simulink library "SCAN"  (R2016a)
settings: Solver=ode45  StartTime=0.0  StopTime=10.0  RelTol=1e-3
undefined symbols (not defined in the file): BLOCK_SIZE
settings Model: Creator=oelkawok  LastModifiedBy=oelkawok
settings DataIOCC: LimitDataPoints=on
settings DebuggingCC: AllowSymbolicDim=off

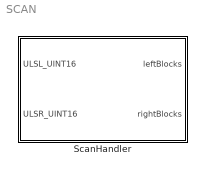
== system SCAN ==
  ScanHandler : Subsystem

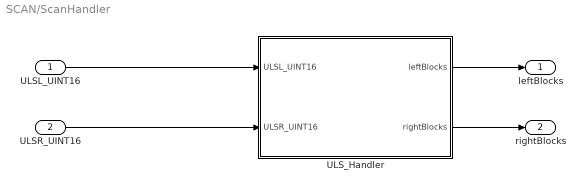
== system SCAN/ScanHandler ==
  ULSL_UINT16 : Inport  OutDataTypeStr=uint16  PortDimensions=1  SampleTime=[0.0050000000000000001,0]
  ULSR_UINT16 : Inport  Port=2  OutDataTypeStr=uint16  PortDimensions=1  SampleTime=[0.0050000000000000001,0]
  ULS_Handler : Subsystem
  leftBlocks : Outport
  rightBlocks : Outport  Port=2
  wires:
  ULSL_UINT16/1 -> ULS_Handler/1(ULSL_UINT16)
  ULSR_UINT16/1 -> ULS_Handler/2(ULSR_UINT16)
  ULS_Handler/1(leftBlocks) -> leftBlocks/1
  ULS_Handler/2(rightBlocks) -> rightBlocks/1

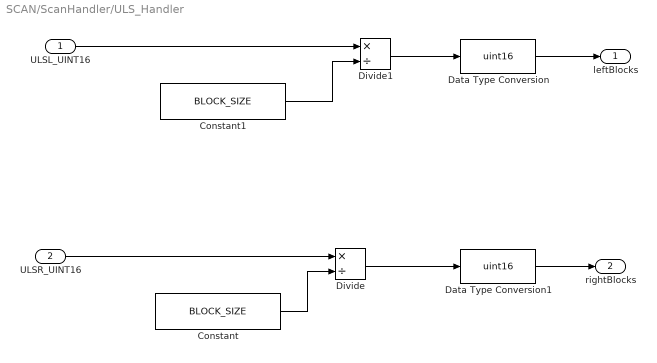
== system SCAN/ScanHandler/ULS_Handler ==
  ULSL_UINT16 : Inport  OutDataTypeStr=uint16  PortDimensions=1  SampleTime=[0.0050000000000000001,0]
  ULSR_UINT16 : Inport  Port=2  OutDataTypeStr=uint16  PortDimensions=1  SampleTime=[0.0050000000000000001,0]
  Constant : Constant  Value=BLOCK_SIZE
  Constant1 : Constant  Value=BLOCK_SIZE
  Data Type Conversion : DataTypeConversion  OutDataTypeStr=uint16
  Data Type Conversion1 : DataTypeConversion  OutDataTypeStr=uint16
  Divide : Product  Inputs=*/
  Divide1 : Product  Inputs=*/
  leftBlocks : Outport
  rightBlocks : Outport  Port=2
  wires:
  ULSR_UINT16/1 -> Divide/1
  Constant/1 -> Divide/2
  ULSL_UINT16/1 -> Divide1/1
  Constant1/1 -> Divide1/2
  Divide/1 -> Data Type Conversion1/1
  Divide1/1 -> Data Type Conversion/1
  Data Type Conversion/1 -> leftBlocks/1
  Data Type Conversion1/1 -> rightBlocks/1
